simulink model "CL_sim"  (Simulink 7.3)
settings: Solver=ode45  StartTime=0  StopTime=404  RelTol=1e-3
undefined symbols (not defined in the file or in its folder): Abo, Bbo, PQ, Tsd, Tss
settings Model: Creator=peteryoung  LastModifiedBy=youngpc  ExtModeAutoUpdateStatusClock=off
settings OptimizationCC: InitFltsAndDblsToZero=on
settings DebuggingCC: SaveWithParameterizedLinksMsg=none  SignalResolutionControl=TryResolveAllWithWarning  MultiTaskDSMMsg=warning  MultiTaskCondExecSysMsg=none
settings RTWCC: IncludeERTFirstTime=on
settings GRTTargetCC: TargetFcnLib=ansi_tfl_tmw.mat

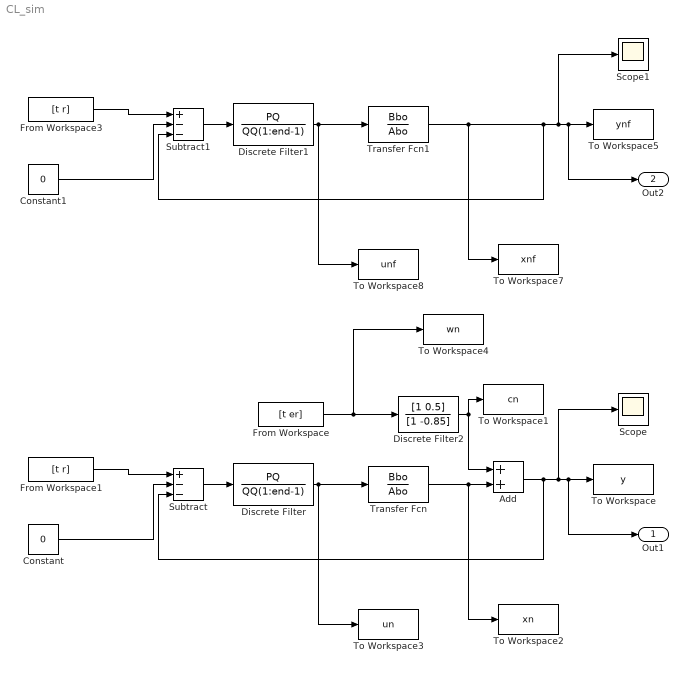
== system CL_sim ==
  Add : Sum  OutDataType=sfix(16)  OutScaling=2^-10
  Constant : Constant  Value=0  OutDataType=sfix(16)  OutScaling=2^0
  Constant1 : Constant  Value=0  OutDataType=sfix(16)  OutScaling=2^0
  Discrete Filter : DiscreteFilter  Numerator=PQ  Denominator=QQ(1:end-1)  SampleTime=Tsd
  Discrete Filter1 : DiscreteFilter  Numerator=PQ  Denominator=QQ(1:end-1)  SampleTime=Tsd
  Discrete Filter2 : DiscreteFilter  Numerator=[1 0.5]  Denominator=[1 -0.85]  SampleTime=Tss
  From Workspace : FromWorkspace  VariableName=[t er]  SampleTime=Tss
  From Workspace1 : FromWorkspace  VariableName=[t r]  SampleTime=Tss
  From Workspace3 : FromWorkspace  VariableName=[t r]  SampleTime=Tss
  Scope : Scope
  Scope1 : Scope
  Subtract : Sum  Inputs=+--  OutDataType=sfix(16)  OutScaling=2^-10
  Subtract1 : Sum  Inputs=+--  OutDataType=sfix(16)  OutScaling=2^-10
  To Workspace : ToWorkspace  VariableName=y  SampleTime=Tss  SaveFormat=Array
  To Workspace1 : ToWorkspace  VariableName=cn  SampleTime=Tss  SaveFormat=Array
  To Workspace2 : ToWorkspace  VariableName=xn  SampleTime=Tss  SaveFormat=Array
  To Workspace3 : ToWorkspace  VariableName=un  SampleTime=Tss  SaveFormat=Array
  To Workspace4 : ToWorkspace  VariableName=wn  SampleTime=Tss  SaveFormat=Array
  To Workspace5 : ToWorkspace  VariableName=ynf  SampleTime=Tss  SaveFormat=Array
  To Workspace7 : ToWorkspace  VariableName=xnf  SampleTime=Tss  SaveFormat=Array
  To Workspace8 : ToWorkspace  VariableName=unf  SampleTime=Tss  SaveFormat=Array
  Transfer Fcn : TransferFcn  Numerator=Bbo  Denominator=Abo
  Transfer Fcn1 : TransferFcn  Numerator=Bbo  Denominator=Abo
  Out1 : Outport  OutDataType=sfix(16)  OutScaling=2^0
  Out2 : Outport  Port=2  OutDataType=sfix(16)  OutScaling=2^0
  wires:
  Subtract/1 -> Discrete Filter/1
  Discrete Filter/1 -> To Workspace3/1, Transfer Fcn/1
  Transfer Fcn/1 -> Add/2, To Workspace2/1
  Discrete Filter2/1 -> Add/1, To Workspace1/1
  Add/1 -> Scope/1, To Workspace/1, Out1/1, Subtract/3
  Constant/1 -> Subtract/2
  From Workspace/1 -> Discrete Filter2/1, To Workspace4/1
  From Workspace1/1 -> Subtract/1
  Subtract1/1 -> Discrete Filter1/1
  Discrete Filter1/1 -> To Workspace8/1, Transfer Fcn1/1
  Transfer Fcn1/1 -> To Workspace7/1, Scope1/1, To Workspace5/1, Out2/1, Subtract1/3
  Constant1/1 -> Subtract1/2
  From Workspace3/1 -> Subtract1/1
